simulink library "wnnsources"  (R2021b)
settings: Solver=VariableStepAuto  StartTime=0.0  StopTime=10.0  RelTol=1e-3
undefined symbols (not defined in the file or in its folder): matdChol
settings Model: Creator=20214358  LastModifiedBy=20214358

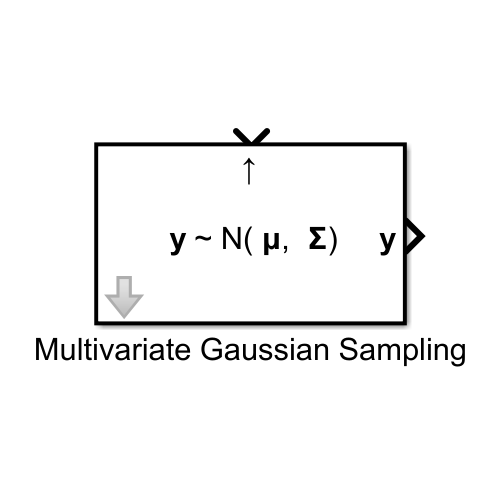
[thumbnail: Simulink's stored preview of the top-level diagram]
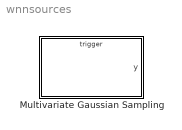
== system wnnsources ==
  Multivariate Gaussian Sampling : Subsystem  mask{vecdAvg=[1 1], matdCov=[2 1; 1 2], nSeed=0}
      mask prompts: vecdAvg "Average Vector"; matdCov "Covariance Matrix"; nSeed "Seed"
      mask init:
      | % Get number of dimensions
      | nDims=length(vecdAvg);
      | [nDims1, nDims2] = size(matdCov);
      | 
      | % Check number of dimensions
      | if nDims1 ~= nDims || nDims2 ~= nDims
      |     error('Covariance matrix and average vector dimensions are not compatible');
      | end
      | 
      | % Compute Cholesky decomposition of the covariance matrix
      | [matdChol,flag] = chol(matdCov)
      | 
      | % Check whether the covariance matrix is positive definite
      | if flag ~= 0
      |     error('Covariance matrix is not symmetric positive definite.');
      | end
      | 
      | % Initialize seeds along dimensions
      | nSeeds = [1:nDims]+nSeed;
      mask Display:
      | disp('{\bf y} \sim N({\bf \mu}, {\bf \Sigma})','interpreter','tex');
      | port_label('output', 1,'{\bf y}','interpreter','tex')
      | port_label('trigger','\uparrow','interpreter','tex')

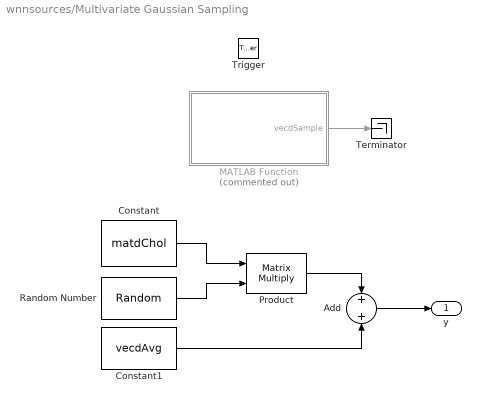
== system wnnsources/Multivariate Gaussian Sampling ==
  Trigger : TriggerPort  VariantControl=(inherit)  PortDimensions=1
  Add : Sum
  Constant : Constant  Value=matdChol  VectorParams1D=off
  Constant1 : Constant  Value=vecdAvg
  MATLAB Function : MATLAB Function  Commented=on  TreatAsAtomicUnit=on
  Product : Product  Multiplication=Matrix(*)
  Random Number : RandomNumber  Seed=nSeeds
  Terminator : Terminator
  y : Outport
  wires:
  Constant/1 -> Product/1
  Product/1 -> Add/1
  Random Number/1 -> Product/2
  Constant1/1 -> Add/2
  Add/1 -> y/1
  MATLAB Function/1(vecdSample) -> Terminator/1

== matlab function wnnsources/Multivariate Gaussian Sampling/MATLAB Function ==
  data: vecdSample output; vecdAvg parameter; matdCov parameter; nSeed parameter; nDims parameter
function vecdSample = fcn(vecdAvg, matdCov, nSeed, nDims)

% Extrinsic Matlab functions
coder.extrinsic('mvnrnd','rng');

% Persistent variables
persistent bInit

% Initialization
if isempty(bInit)
    rng(nSeed);  
    bInit = 1;
end

% Preallocate output
vecdSample = zeros(1, nDims);

% Draw a sample from a multivariate Gaussian distribution
vecdSample = mvnrnd(vecdAvg, matdCov);
